simulink subsystem "G"  (R2024a)
settings: Solver=VariableStepAuto  StartTime=0.0  StopTime=100.0  RelTol=1e-3
settings Model: DefaultTestHarness=G_Harness1  Creator=nevil  LastModifiedBy=nevil

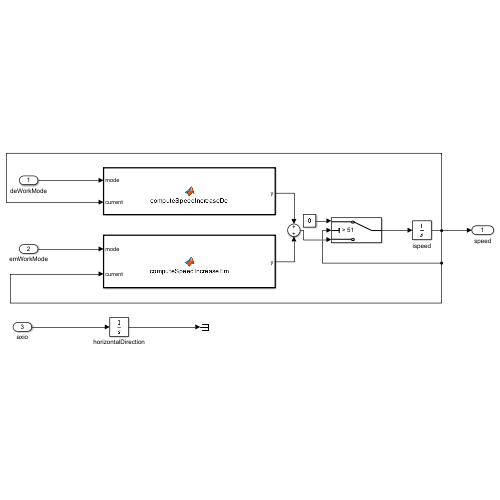
[thumbnail: Simulink's stored preview of the top-level diagram]
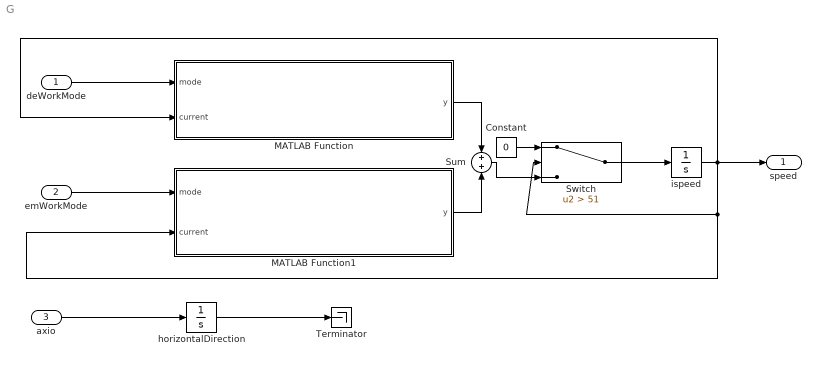
== system G ==
  deWorkMode : Inport
  emWorkMode : Inport  Port=2
  axio : Inport  Port=3
  Constant : Constant  Value=0
  MATLAB Function : MATLAB Function  TreatAsAtomicUnit=on
  MATLAB Function1 : MATLAB Function  TreatAsAtomicUnit=on
  Sum : Sum  Inputs=+|+
  Switch : Switch  Criteria=u2 > Threshold  Threshold=51  SaturateOnIntegerOverflow=off  InputSameDT=off
  Terminator : Terminator
  horizontalDirection : Integrator
  ispeed : Integrator
  speed : Outport
  wires:
  deWorkMode/1 -> MATLAB Function/1(mode)
  axio/1 -> horizontalDirection/1
  horizontalDirection/1 -> Terminator/1
  emWorkMode/1 -> MATLAB Function1/1(mode)
  MATLAB Function1/1(y) -> Sum/2
  MATLAB Function/1(y) -> Sum/1
  ispeed/1 -> Switch/2, MATLAB Function1/2(current), speed/1, MATLAB Function/2(current)
  Sum/1 -> Switch/3
  Switch/1 -> ispeed/1
  Constant/1 -> Switch/1

== matlab function G/MATLAB Function ==
  data: mode input; y output; current input
function y = computeSpeedIncreaseDe(mode, current)
    limitSpeed = 0;
    
    switch(mode)
        case 0
            limitSpeed = 32;
        case 1
            limitSpeed = 28;
        case 2
            limitSpeed = 24;
        case 3
            limitSpeed = 18;
        case 4
            limitSpeed = 6;
        case 5
            limitSpeed = 0;
        case 6
            limitSpeed = 0;
        case 7
            limitSpeed = -10;
        case 8
            limitSpeed = -14;
        case 9
            limitSpeed = -18;
        case 10
            limitSpeed = -20;
        otherwise
            error('Invalid mode');
    end

    if(current + 2 < limitSpeed)
        y = 2;
    else
        y = limitSpeed;
    end
end

== matlab function G/MATLAB Function1 ==
  data: mode input; y output; current input
function y = computeSpeedIncreaseEm(mode, current)
    limitSpeed = 0;
    
    switch(mode)
        case 0
            limitSpeed = 19;
        case 1
            limitSpeed = 16;
        case 2
            limitSpeed = 13;
        case 3
            limitSpeed = 10;
        case 4
            limitSpeed = 6;
        case 5
            limitSpeed = 0;
        case 6
            limitSpeed = 0;
        case 7
            limitSpeed = -9;
        case 8
            limitSpeed = -12;
        case 9
            limitSpeed = -14;
        case 10
            limitSpeed = -16;
        otherwise
            error('Invalid mode');
    end

    if(current + 2 < limitSpeed)
        y = 2;
    else
        y = limitSpeed;
    end
end
